simulink model "AUAV_V3_TestSensors"  (R2015a)
settings: Solver=FixedStepDiscrete  StartTime=0.0  StopTime=10.0  FixedStep=T  RelTol=1e-3
PreLoadFcn:
  | %T = 0.0025;
  | MavlinkBus;
  | mcuInit;
  | % Baro Altitude Computation
  | % =========================
  | basePressure = 98192.64;
  | baseTemp = 288.215;
  | lapseRate = -0.00198122;
  | baseHeight = 0;
undefined symbols (not defined in the file): A0, A14, A15, A2, A3, A4, A5, A6, accBiasRateLimit, apSampleTime, B0, bankCommandLimit, barAdjust, baroCutoff, baroCutTemp, baroOffset, baroScale, barTGain1, barTGain2, barTMean1, barTMean2, bda, bde, bdr, bdt, bICda, bICde, bICdr, bICdt, cubeAccelGain16405, cubeGyroGain16405, cubeMagGain16405, D0, D11, D7, D8, daLimit, data, daTrimMax, daTrimMin, deLimit, derivativesConstant, deTrimMax, deTrimMin, drLimit, drTrimMax, drTrimMin, dtLimit, dtTrimMax, dtTrimMin, F2, F3, G0, G13, G15, gaind, GS_location, gyroBiasRateLimit, IC1max, imuOffset_xacc ... (+77)
libraries: MCHP_Blockset x158, simulink x84, SLUGS_Library x31, aerolibconvert2 x6, aerolibutil x4, aerolibtransform2 x3, dspmtrx3 x2, aerolibobsolete x2
(part 20 of 23)

== system AUAV_V3_TestSensors/Inner Loop// Navigation/Longitudinal Channel Encaps [updated 4.28.16]/Longitudinal Channel/Height Error to Pitch Command [PI]/Trapezoidal Integrator ==
  x : Inport
  Reset : Inport  Port=2
  Constant : Constant  Value=1/3  OutDataTypeStr=single
  Constant1 : Constant  Value=4/3  OutDataTypeStr=single
  Constant2 : Constant  Value=T/2  OutDataTypeStr=single
  Constant3 : Constant  Value=1/3  OutDataTypeStr=single
  Constant5 : Constant  Value=0  OutDataTypeStr=single
  Integer Delay : Delay  DelayLength=1  InputProcessing=Inherited  SampleTime=T
  Integer Delay1 : Delay  InputProcessing=Inherited  SampleTime=T
  Integer Delay2 : Delay  DelayLength=1  InputProcessing=Inherited  SampleTime=T
  Product{,1..3} (4 alike) : Product  OutDataTypeStr=single  RndMeth=Zero
  Protect NaNs : Subsystem
  "Protect NaNs " : Subsystem
  Subtract : Sum  Inputs=3  OutDataTypeStr=single
  Subtract1 : Sum  Inputs=2  OutDataTypeStr=single
  Switch1 : Switch  Criteria=u2 > Threshold  Threshold=0.3  SampleTime=.01
  Int(x) : Outport
  wires:
  Constant/1 -> Product/2
  Constant1/1 -> Product1/2
  Integer Delay/1 -> Product1/1
  Integer Delay1/1 -> Product2/1
  Constant3/1 -> Product2/2
  x/1 -> "Protect NaNs "/1(In1)
  Product/1 -> Subtract/1
  Product1/1 -> Subtract/2
  Product2/1 -> Subtract/3
  Constant2/1 -> Product3/1
  Subtract/1 -> Product3/2
  Subtract1/1 -> Switch1/3
  Integer Delay2/1 -> Subtract1/1
  Product3/1 -> Subtract1/2
  Constant5/1 -> Switch1/1
  Reset/1 -> Switch1/2
  Switch1/1 -> Protect NaNs/1(In1)
  Protect NaNs/1(Out1) -> Int(x)/1, Integer Delay2/1
  "Protect NaNs "/1(Out1) -> Product/1, Integer Delay/1, Integer Delay1/1

== system AUAV_V3_TestSensors/Inner Loop// Navigation/Longitudinal Channel Encaps [updated 4.28.16]/Longitudinal Channel/Pitch To Elevator [PID]/Trapezoidal Integrator ==
  x : Inport
  Reset : Inport  Port=2
  Constant : Constant  Value=1/3  OutDataTypeStr=single
  Constant1 : Constant  Value=4/3  OutDataTypeStr=single
  Constant2 : Constant  Value=T/2  OutDataTypeStr=single
  Constant3 : Constant  Value=1/3  OutDataTypeStr=single
  Constant5 : Constant  Value=0  OutDataTypeStr=single
  Integer Delay : Delay  DelayLength=1  InputProcessing=Inherited  SampleTime=T
  Integer Delay1 : Delay  InputProcessing=Inherited  SampleTime=T
  Integer Delay2 : Delay  DelayLength=1  InputProcessing=Inherited  SampleTime=T
  Product{,1..3} (4 alike) : Product  OutDataTypeStr=single  RndMeth=Zero
  "Protect NaNs " : Subsystem
  Protect NaNs1 : Subsystem
  Subtract : Sum  Inputs=3  OutDataTypeStr=single
  Subtract1 : Sum  Inputs=2  OutDataTypeStr=single
  Switch1 : Switch  Criteria=u2 > Threshold  Threshold=0.3  SampleTime=.01
  Int(x) : Outport
  wires:
  Switch1/1 -> Protect NaNs1/1(In1)
  Reset/1 -> Switch1/2
  Constant5/1 -> Switch1/1
  Product3/1 -> Subtract1/2
  Integer Delay2/1 -> Subtract1/1
  Subtract1/1 -> Switch1/3
  Subtract/1 -> Product3/2
  Constant2/1 -> Product3/1
  Product2/1 -> Subtract/3
  Product1/1 -> Subtract/2
  Product/1 -> Subtract/1
  x/1 -> "Protect NaNs "/1(In1)
  Constant3/1 -> Product2/2
  Integer Delay1/1 -> Product2/1
  Integer Delay/1 -> Product1/1
  Constant1/1 -> Product1/2
  Constant/1 -> Product/2
  Protect NaNs1/1(Out1) -> Integer Delay2/1, Int(x)/1
  "Protect NaNs "/1(Out1) -> Integer Delay1/1, Integer Delay/1, Product/1

== system AUAV_V3_TestSensors/Inner Loop// Navigation/Longitudinal Channel Encaps [updated 4.28.16]/Longitudinal Channel/Pitot Control End/ 0.3 sec tau for high speeds ==
  In1 : Inport
  Constant : Constant  Value=T
  Constant1 : Constant  Value=f
  Embedded MATLAB Function : MATLAB Function  TreatAsAtomicUnit=on
  Out1 : Outport
  wires:
  Constant/1 -> Embedded MATLAB Function/2(T)
  Constant1/1 -> Embedded MATLAB Function/3(f)
  Embedded MATLAB Function/1(y) -> Out1/1
  In1/1 -> Embedded MATLAB Function/1(u)

== system AUAV_V3_TestSensors/Inner Loop// Navigation/Longitudinal Channel Encaps [updated 4.28.16]/Longitudinal Channel/Pitot Control End/Air Density from Height ==
  h(m) : Inport
  Add : Sum  Inputs=+-
  Constant : Constant  OutDataTypeStr=single
  Constant 2 from Model : Constant  Value=4.255876  OutDataTypeStr=single
  Constant from Model : Constant  Value=145442  OutDataTypeStr=single
  Divide : Product  Inputs=*/
  Divide1 : Product
  Length Conversion : aerolibconvert2/Length Conversion  IU=m  OU=ft
  Rho_0 (Kg/m^3) : Constant  Value=1.225  OutDataTypeStr=single
  "[0 1000]" : Saturate  UpperLimit=1000  LowerLimit=0
  dsPIC Power : Subsystem  AncestorBlock=SLUGS_Library/dsPIC Power
  rho (Kg/m^3) : Outport
  wires:
  Constant/1 -> Add/1
  Divide/1 -> Add/2
  h(m)/1 -> "[0 1000]"/1
  Constant from Model/1 -> Divide/2
  Rho_0 (Kg/m^3)/1 -> Divide1/2
  Divide1/1 -> rho (Kg/m^3)/1
  Length Conversion/1 -> Divide/1
  Add/1 -> dsPIC Power/1(u)
  Constant 2 from Model/1 -> dsPIC Power/2(v)
  dsPIC Power/1(u^v) -> Divide1/1
  "[0 1000]"/1 -> Length Conversion/1

== system AUAV_V3_TestSensors/Inner Loop// Navigation/Longitudinal Channel Encaps [updated 4.28.16]/Longitudinal Channel/Pitot Control End/Compute Airspeed ==
  Dyn P : Inport
  rho : Inport  Port=2
  Divide2 : Product  Inputs=**/
  "[ 0.01 50000]" : Saturate  UpperLimit=50000  LowerLimit=0.01
  a : Constant  Value=2  OutDataTypeStr=single
  dsPIC_SQRT : Subsystem  AncestorBlock=SLUGS_Library/dsPIC_SQRT
  Airspeed m(s) : Outport
  wires:
  "[ 0.01 50000]"/1 -> Divide2/3
  rho/1 -> "[ 0.01 50000]"/1
  Dyn P/1 -> Divide2/2
  a/1 -> Divide2/1
  dsPIC_SQRT/1(sqrt(x)) -> Airspeed m(s)/1
  Divide2/1 -> dsPIC_SQRT/1(x)

== system AUAV_V3_TestSensors/Inner Loop// Navigation/Longitudinal Channel Encaps [updated 4.28.16]/Longitudinal Channel/Pitot Control End/Protect NaN ==
  In1 : Inport
  Integer Delay3 : Delay  DelayLength=1  InputProcessing=Inherited  SampleTime=T
  Relational Operator2 : RelationalOperator  Operator===  OutDataTypeStr=uint(8)
  Switch3 : Switch  Criteria=u2 > Threshold  Threshold=0.3  SampleTime=.01
  Out1 : Outport
  wires:
  Integer Delay3/1 -> Switch3/3
  Switch3/1 -> Out1/1, Integer Delay3/1
  In1/1 -> Relational Operator2/2, Relational Operator2/1, Switch3/1
  Relational Operator2/1 -> Switch3/2

== system AUAV_V3_TestSensors/Inner Loop// Navigation/Navigation Encaps [updated 4.28.16]/Navigation/Circle Navigation/Get SP Location ==
  GS LLA : Inport
  GS R_in : Inport  Port=2
  ISR Location : Inport  Port=3
  Demux : Demux  Outputs=3
  Geod2LTP : SLUGS_Library/Navigation/Geod2LTP
  Integer Delay1 : Delay  DelayLength=1  InputProcessing=Inherited
  Selector : Selector  InputPortWidth=3  Indices=[3]
  Zero out Z2 : MATLAB Function  TreatAsAtomicUnit=on
  Hc : Outport
  SP : Outport  Port=2
  wires:
  Integer Delay1/1 -> Hc/1
  Selector/1 -> Integer Delay1/1
  Zero out Z2/1(P) -> SP/1
  Geod2LTP/1 -> Selector/1, Zero out Z2/1(Pin)
  GS LLA/1 -> Geod2LTP/1
  Demux/3 -> Geod2LTP/5
  Demux/2 -> Geod2LTP/4
  Demux/1 -> Geod2LTP/3
  GS R_in/1 -> Geod2LTP/2
  ISR Location/1 -> Demux/1

== system AUAV_V3_TestSensors/Inner Loop// Navigation/Navigation Encaps [updated 4.28.16]/Navigation/Circle Navigation/Inside the Circle, Keep Straight until intersection ==
  ISR Loc : Inport
  R : Inport  Port=2
  Puav : Inport  Port=3
  Action Port : ActionPort  ActionType=elseif
  Compute Head of Circle : MATLAB Function  TreatAsAtomicUnit=on
  RTB1 : Constant  OutDataTypeStr=uint8
  Subtract : Sum  Inputs=+-  OutDataTypeStr=single
  L2 Vec : Outport
  Mode : Outport  Port=2
  wires:
  RTB1/1 -> Mode/1
  R/1 -> Compute Head of Circle/1(R)
  ISR Loc/1 -> Compute Head of Circle/2(ISR)
  Compute Head of Circle/1(topCoord) -> Subtract/1
  Puav/1 -> Subtract/2
  Subtract/1 -> L2 Vec/1

== system AUAV_V3_TestSensors/Inner Loop// Navigation/Navigation Encaps [updated 4.28.16]/Navigation/Circle Navigation/Intersection. Circular Navigation ==
  R : Inport
  L2 : Inport  Port=2
  d : Inport  Port=3
  ISR Loc : Inport  Port=4
  UAV m ISR : Inport  Port=5
  Vxyz : Inport  Port=6
  |Vg| : Inport  Port=7
  Puav : Inport  Port=8
  Action Port : ActionPort  ActionType=else
  Compute Angle Between Vectors1 : Subsystem  AncestorBlock=SLUGS_Library/Compute Angle Between Vectors
  Compute Angle Between Vectors2 : Subsystem  AncestorBlock=SLUGS_Library/Compute Angle Between Vectors
  Embedded MATLAB Function : MATLAB Function  TreatAsAtomicUnit=on
  Product{,1..2,4..5,7} (6 alike) : Product  RndMeth=Zero
  Product3 : Product  Inputs=*/  RndMeth=Zero
  Product6 : Product  Inputs=*/  RndMeth=Zero
  RTB1 : Constant  Value=2  OutDataTypeStr=uint8
  Relational Operator : RelationalOperator  Operator=<=  OutDataTypeStr=boolean
  Subtract : Sum  Inputs=+-+
  Subtract1 : Sum  Inputs=2
  Subtract2 : Sum  Inputs=+-
  Subtract3 : Sum  Inputs=2
  Subtract5 : Sum  Inputs=+-
  Subtract6 : Sum  Inputs=-+
  Switch1 : Switch  Criteria=u2 > Threshold  Threshold=0.3  ZeroCross=off
  "d " : InportShadow  Port=3
  dsPIC_ABS : Subsystem  AncestorBlock=SLUGS_Library/dsPIC_ABS
  dsPIC_ABS1 : Subsystem  AncestorBlock=SLUGS_Library/dsPIC_ABS
  dsPIC_SQRT : Subsystem  AncestorBlock=SLUGS_Library/dsPIC_SQRT
  negprotect1 : MATLAB Function  TreatAsAtomicUnit=on
  negprotect2 : MATLAB Function  TreatAsAtomicUnit=on
  L2 Vec : Outport
  Mode : Outport  Port=2
  wires:
  R/1 -> Product/1, Product/2
  L2/1 -> Product1/1, Product1/2
  d/1 -> Product2/1, Product2/2, Subtract1/1, Subtract1/2
  Product/1 -> Subtract/1, Subtract2/1  "r^2"
  Product1/1 -> Subtract/2
  Product2/1 -> Subtract/3
  Subtract/1 -> Product3/1  "r^2 - L2^2 + d^2"
  negprotect2/1(zpVal) -> Product3/2  "2d"
  Subtract1/1 -> negprotect2/1(val)
  Product3/1 -> Product4/2, Product4/1, [a]  "a"
  Product4/1 -> Subtract2/2  "a^2"
  Subtract2/1 -> dsPIC_SQRT/1(x)  "h"
  negprotect1/1(zpVal) -> Product6/2  "d"
  "d "/1 -> negprotect1/1(val)
  ISR Loc/1 -> Subtract3/1
  Subtract3/1 -> Embedded MATLAB Function/2(P2)  "P2"
  UAV m ISR/1 -> Product6/1
  Product7/1 -> Subtract3/2
  Product6/1 -> Product7/1, [UavMIsDbd]
  [a] -> Product7/2
  [UavMIsDbd] -> Product5/2
  Vxyz/1 -> Compute Angle Between Vectors1/1(Vxyz), Compute Angle Between Vectors2/1(Vxyz)
  |Vg|/1 -> Compute Angle Between Vectors1/2(|Vg|), Compute Angle Between Vectors2/2(|Vg|)
  Compute Angle Between Vectors2/1(alpha) -> dsPIC_ABS1/1(x)
  dsPIC_ABS1/1(|x|) -> Relational Operator/1
  Compute Angle Between Vectors1/1(alpha) -> dsPIC_ABS/1(x)
  dsPIC_ABS/1(|x|) -> Relational Operator/2
  Relational Operator/1 -> Switch1/2
  RTB1/1 -> Mode/1
  dsPIC_SQRT/1(sqrt(x)) -> Product5/1  "h"
  Product5/1 -> Embedded MATLAB Function/1(hFact)
  Subtract5/1 -> Compute Angle Between Vectors2/3(P3), Switch1/1
  Embedded MATLAB Function/1(P31) -> Subtract5/1
  Subtract6/1 -> Compute Angle Between Vectors1/3(P3), Switch1/3
  Embedded MATLAB Function/2(P32) -> Subtract6/2
  Puav/1 -> Subtract5/2, Subtract6/1
  Switch1/1 -> L2 Vec/1

== system AUAV_V3_TestSensors/Inner Loop// Navigation/Navigation Encaps [updated 4.28.16]/Navigation/Circle Navigation/No intersection, Navigate to ISR ==
  Puav : Inport
  ISR Loc : Inport  Port=2
  Action Port : ActionPort  ActionType=then
  RTB1 : Constant  Value=0  OutDataTypeStr=uint8
  Subtract : Sum  Inputs=+-
  L2 Vec : Outport
  Mode : Outport  Port=2
  wires:
  ISR Loc/1 -> Subtract/1
  Puav/1 -> Subtract/2
  Subtract/1 -> L2 Vec/1
  RTB1/1 -> Mode/1

== system AUAV_V3_TestSensors/Inner Loop// Navigation/Navigation Encaps [updated 4.28.16]/Navigation/Circle Navigation/Vector Norm ==
  Vector : Inport
  dsPIC Dot Product : SLUGS_Library/dsPIC Dot Product
  dsPIC_SQRT : Subsystem  AncestorBlock=SLUGS_Library/dsPIC_SQRT
  Norm : Outport
  wires:
  dsPIC_SQRT/1(sqrt(x)) -> Norm/1
  Vector/1 -> dsPIC Dot Product/2, dsPIC Dot Product/1
  dsPIC Dot Product/1 -> dsPIC_SQRT/1(x)

== system AUAV_V3_TestSensors/Inner Loop// Navigation/Navigation Encaps [updated 4.28.16]/Navigation/Circle Navigation/dsPIC_ABS ==
  x : Inport
  Abs : Abs
  Environment Controller : simulink/Signal Routing/Environment Controller
  myAbs() apUtils.c [updated 5.1.16] : MCHP_Blockset/User Functions/C Function Call  ParseFilesChkbx=off  ListFunctions1=Custom Function  Function1=float myAbs(float x)  AddHeaderDeclaration=off  Function1Type=when block is updated (default)  Fct1BlockIn=x  FctReturnBlockOut=on  DataCollected=0  ORDERING=None  SampleTime=-1  MCHP_MASTERLINK=|  PinDigitalInput=[]  PinDigitalOutput=[]  PinAnalogInput=[]
      | AUAV_V3_TestSensors/Microchip Master
      | AUAV V3 Board
      | Busy Flag on D2 (RA6)
  |x| : Outport
  wires:
  Environment Controller/1 -> |x|/1
  Abs/1 -> Environment Controller/1
  myAbs() apUtils.c [updated 5.1.16]/1 -> Environment Controller/2
  x/1 -> Abs/1, myAbs() apUtils.c [updated 5.1.16]/1

== system AUAV_V3_TestSensors/Inner Loop// Navigation/Navigation Encaps [updated 4.28.16]/Navigation/Get 2D Groundspeed/Vector Norm ==
  Vector : Inport
  dsPIC Dot Product : SLUGS_Library/dsPIC Dot Product
  dsPIC_SQRT : Subsystem  AncestorBlock=SLUGS_Library/dsPIC_SQRT
  Norm : Outport
  wires:
  dsPIC_SQRT/1(sqrt(x)) -> Norm/1
  Vector/1 -> dsPIC Dot Product/2, dsPIC Dot Product/1
  dsPIC Dot Product/1 -> dsPIC_SQRT/1(x)

== system AUAV_V3_TestSensors/Inner Loop// Navigation/Navigation Encaps [updated 4.28.16]/Navigation/L2+/Get Sin, Cos eta ==
  |V_g| : Inport
  L2_vec : Inport  Port=2
  Vxyz : Inport  Port=3
  "2D Dot Product " : Subsystem
  Compare To Zero : simulink/Logic and Bit Operations/Compare To Zero  relop===  OutDataTypeStr=uint8  ZeroCross=off
  Dead Zone : DeadZone  LowerValue=-0.1  UpperValue=0.1  SaturateOnIntegerOverflow=on
  Display : Display
  Display1 : Display
  Divide1 : Product  Inputs=/*
  Divide2 : Product  Inputs=*/
  Get Groundspeed : Subsystem
  Get ZProd : Subsystem
  Product1 : Product  RndMeth=Zero
  Switch : Switch  Criteria=u2 > Threshold  Threshold=0.3  ZeroCross=off
  Switch2 : Switch  Criteria=u2 > Threshold  Threshold=0.3  ZeroCross=off
  cos(pi/2) : Constant  Value=0  OutDataTypeStr=single
  negprotect : MATLAB Function  TreatAsAtomicUnit=on
  sin(pi/2) : Constant  OutDataTypeStr=single
  sin(eta) : Outport
  cos(eta) : Outport  Port=2
  wires:
  negprotect/1(zpVal) -> Divide2/2, Divide1/1, Dead Zone/1
  Switch/1 -> Display/1, sin(eta)/1
  Divide2/1 -> Switch/3
  Get ZProd/1(Z_prod) -> Divide2/1
  Divide1/1 -> Switch2/3
  cos(pi/2)/1 -> Switch2/1
  Switch2/1 -> Display1/1, cos(eta)/1
  sin(pi/2)/1 -> Switch/1
  "2D Dot Product "/1(2D _dot) -> Divide1/2
  Product1/1 -> negprotect/1(val)
  |V_g|/1 -> Product1/2
  Get Groundspeed/1(|L2|) -> Product1/1
  Vxyz/1 -> "2D Dot Product "/1(Vxyz), Get ZProd/2(Vxyz)
  L2_vec/1 -> Get Groundspeed/1(L2_vec), "2D Dot Product "/2(L2_vec), Get ZProd/1(L2_vec)
  Dead Zone/1 -> Compare To Zero/1
  Compare To Zero/1 -> Switch2/2, Switch/2

== system AUAV_V3_TestSensors/Inner Loop// Navigation/Navigation Encaps [updated 4.28.16]/Navigation/L2+/L2+ ==
  sin(eta) : Inport
  |V_g| : Inport  Port=2
  T* : Inport  Port=3
  Display3 : Display
  Divide : Product  Inputs=**/
  Gain : Gain  Gain=2  SampleTime=0.01
  negprotect : MATLAB Function  TreatAsAtomicUnit=on
  a_c : Outport
  wires:
  T*/1 -> negprotect/1(val)
  Gain/1 -> Display3/1, a_c/1
  |V_g|/1 -> Divide/2
  Divide/1 -> Gain/1
  sin(eta)/1 -> Divide/1
  negprotect/1(zpVal) -> Divide/3

== system AUAV_V3_TestSensors/Inner Loop// Navigation/Navigation Encaps [updated 4.28.16]/Navigation/L2+/Subsystem ==
  a_c : Inport
  Bank  Limit Command : Saturate  UpperLimit=bankCommandLimit  LowerLimit=-bankCommandLimit  SampleTime=apSampleTime
  Constant : Constant  Value=ISA_g  OutDataTypeStr=single
  Product : Product  Inputs=*/  RndMeth=Zero
  To Workspace3 : ToWorkspace  VariableName=Phic  SampleTime=-1
  dsPIC_atan : Subsystem  AncestorBlock=SLUGS_Library/dsPIC_atan
  phi_c : Outport
  wires:
  Bank  Limit Command/1 -> To Workspace3/1, phi_c/1
  dsPIC_atan/1(atan(x)) -> Bank  Limit Command/1
  Product/1 -> dsPIC_atan/1(x)
  Constant/1 -> Product/2
  a_c/1 -> Product/1

== system AUAV_V3_TestSensors/Inner Loop// Navigation/Navigation Encaps [updated 4.28.16]/Navigation/L2+/dsPIC_ABS ==
  x : Inport
  Abs : Abs
  Environment Controller : simulink/Signal Routing/Environment Controller
  myAbs() apUtils.c [updated 5.1.16] : MCHP_Blockset/User Functions/C Function Call  ParseFilesChkbx=off  ListFunctions1=Custom Function  Function1=float myAbs(float x)  AddHeaderDeclaration=on  Function1Type=when block is updated (default)  Fct1BlockIn=x  FctReturnBlockOut=on  DataCollected=0  ORDERING=None  SampleTime=-1  MCHP_MASTERLINK=|  PinDigitalInput=[]  PinDigitalOutput=[]  PinAnalogInput=[]
      | AUAV_V3_TestSensors/Microchip Master
      | AUAV V3 Board
      | Busy Flag on D2 (RA6)
  |x| : Outport
  wires:
  Environment Controller/1 -> |x|/1
  Abs/1 -> Environment Controller/1
  myAbs() apUtils.c [updated 5.1.16]/1 -> Environment Controller/2
  x/1 -> Abs/1, myAbs() apUtils.c [updated 5.1.16]/1

== system AUAV_V3_TestSensors/Inner Loop// Navigation/Navigation Encaps [updated 4.28.16]/Navigation/L2+/dsPIC_atan2 ==
  u : Inport
  v : Inport  Port=2
  Environment Controller : simulink/Signal Routing/Environment Controller
  Trigonometric Function : Trigonometry  Operator=atan2
  myAtan2() apUtils.c [updated 5.1.16] : MCHP_Blockset/User Functions/C Function Call  ParseFilesChkbx=off  ListFunctions1=Custom Function  Function1=float myAtan2(float num, float denom)  AddHeaderDeclaration=on  Function1Type=when block is updated (default)  Fct1BlockIn="num  , denom"  FctReturnBlockOut=on  DataCollected=0  ORDERING=None  SampleTime=-1  MCHP_MASTERLINK=|  PinDigitalInput=[]  PinDigitalOutput=[]  PinAnalogInput=[]
      | AUAV_V3_TestSensors/Microchip Master
      | AUAV V3 Board
      | Busy Flag on D2 (RA6)
  atan2(x,y) : Outport
  wires:
  Environment Controller/1 -> atan2(x,y)/1
  myAtan2() apUtils.c [updated 5.1.16]/1 -> Environment Controller/2
  Trigonometric Function/1 -> Environment Controller/1
  v/1 -> Trigonometric Function/2, myAtan2() apUtils.c [updated 5.1.16]/2
  u/1 -> Trigonometric Function/1, myAtan2() apUtils.c [updated 5.1.16]/1

== system AUAV_V3_TestSensors/Inner Loop// Navigation/Navigation Encaps [updated 4.28.16]/Navigation/L2+/if sin(eta) < 0 - maxAcc else maxAcc  ==
  sin(eta) : Inport
  Compare To Zero : simulink/Logic and Bit Operations/Compare To Zero  relop=<  OutDataTypeStr=uint8  ZeroCross=off
  Constant1 : Constant  Value=maxAcc  OutDataTypeStr=single
  Constant9 : Constant  Value=-maxAcc  OutDataTypeStr=single
  Switch1 : Switch  Criteria=u2 > Threshold  Threshold=0.3
  + - maxAcc : Outport
  wires:
  Switch1/1 -> + - maxAcc/1
  sin(eta)/1 -> Compare To Zero/1
  Constant1/1 -> Switch1/3
  Constant9/1 -> Switch1/1
  Compare To Zero/1 -> Switch1/2

== system AUAV_V3_TestSensors/Inner Loop// Navigation/Navigation Encaps [updated 4.28.16]/Navigation/Line Segment/Vector Norm ==
  Vector : Inport
  dsPIC Dot Product : SLUGS_Library/dsPIC Dot Product
  dsPIC_SQRT : Subsystem  AncestorBlock=SLUGS_Library/dsPIC_SQRT
  Norm : Outport
  wires:
  dsPIC_SQRT/1(sqrt(x)) -> Norm/1
  Vector/1 -> dsPIC Dot Product/2, dsPIC Dot Product/1
  dsPIC Dot Product/1 -> dsPIC_SQRT/1(x)

== system AUAV_V3_TestSensors/Inner Loop// Navigation/Navigation Encaps [updated 4.28.16]/Navigation/Normal WP Navigation/Compute WP Switching Trigger ==
  ToWp : Inport
  T1 : Inport  Port=2
  N1 : Inport  Port=3
  LeadDistance : Inport  Port=4
  Puav : Inport  Port=5
  L2 : Inport  Port=6
  Add : Sum  Inputs=+-
  Add1 : Sum  Inputs=+-
  Add3 : Sum  Inputs=--
  Compute Projection : Subsystem
  Constant1 : Constant  Value=0  OutDataTypeStr=single
  Constant3 : Constant  Value=MaxDwnPthStar  OutDataTypeStr=single
  Constant4 : Constant  Value=tanIntercept  OutDataTypeStr=single
  Divide : Product  Inputs=*/
  Divide1 : Product
  Product : Product  RndMeth=Zero
  Product1 : Product  RndMeth=Zero
  Product2 : Product  RndMeth=Zero
  "Puav " : InportShadow  Port=5
  Relational Operator : RelationalOperator  Operator=>  OutDataTypeStr=boolean
  Subtract : Sum  Inputs=+-  OutDataTypeStr=single
  Switch Distance Less than? : RelationalOperator  Operator=<  OutDataTypeStr=uint(8)  SampleTime=apSampleTime
  Switch1 : Switch  Criteria=u2 > Threshold  Threshold=0.3
  "T1 " : InportShadow  Port=2
  "WP1 " : InportShadow
  dsPIC Dot Product : SLUGS_Library/dsPIC Dot Product
  dsPIC_ABS : Subsystem  AncestorBlock=SLUGS_Library/dsPIC_ABS
  dsPIC_SQRT : Subsystem  AncestorBlock=SLUGS_Library/dsPIC_SQRT
  max : SLUGS_Library/max
  max1 : SLUGS_Library/max
  min : SLUGS_Library/min
  Switch : Outport
  Dist2WP1 : Outport  Port=2
  L2Vec : Outport  Port=3
  wires:
  Puav/1 -> Compute Projection/1(Pned)
  Compute Projection/1(D2wp1) -> Switch Distance Less than?/1, Dist2WP1/1, [Dwp1]
  LeadDistance/1 -> Switch Distance Less than?/2
  ToWp/1 -> Compute Projection/2(ToWp)
  T1/1 -> Compute Projection/3(T)
  Switch Distance Less than?/1 -> Switch/1
  "Puav "/1 -> Subtract/1
  "WP1 "/1 -> Subtract/2
  Subtract/1 -> dsPIC Dot Product/1, [Pwp1]
  dsPIC Dot Product/1 -> dsPIC_ABS/1(x)  "e_N"
  dsPIC_ABS/1(|x|) -> Divide/1, [abs_e_N]
  Constant4/1 -> Divide/2
  Divide/1 -> min/2  "|e_N|/tanInt"
  L2/1 -> Divide1/1, [L2]
  Constant3/1 -> Divide1/2
  Divide1/1 -> min/1
  min/1 -> max1/1, Switch1/1  "minDownPath"
  Relational Operator/1 -> Switch1/2
  [L2] -> Relational Operator/2
  [abs_e_N] -> Relational Operator/1
  Switch1/1 -> Add1/2  "L2DownPath"
  Add/1 -> dsPIC_SQRT/1(x)
  dsPIC_SQRT/1(sqrt(x)) -> max1/2
  [L2] -> Product/1, Product/2
  Product/1 -> Add/1
  [abs_e_N] -> Product1/2, Product1/1
  Product1/1 -> Add/2
  max1/1 -> Switch1/3
  [Dwp1] -> Add1/1
  Add1/1 -> max/1
  Constant1/1 -> max/2
  max/1 -> Product2/1
  "T1 "/1 -> Product2/2
  Product2/1 -> Add3/1
  [Pwp1] -> Add3/2
  Add3/1 -> L2Vec/1
  N1/1 -> dsPIC Dot Product/2

== system AUAV_V3_TestSensors/Inner Loop// Navigation/Navigation Encaps [updated 4.28.16]/Navigation/Normal WP Navigation/Get Frenet ==
  GS LLA : Inport
  GS R_in : Inport  Port=2
  From WP : Inport  Port=3
  To WP : Inport  Port=4
  TurnLeadTime : Inport  Port=5
  |V_g| : Inport  Port=6
  Enable : EnablePort
  Compute Frenet : Subsystem  AncestorBlock=SLUGS_Library/Navigation/Compute Frenet
  Demux1 : Demux  Outputs=3
  GS LLA_1 : InportShadow
  GS R_in_1 : InportShadow  Port=2
  Integer Delay1 : Delay  DelayLength=1  InitialCondition=1  InputProcessing=Inherited
  Product1 : Product  OutDataTypeStr=single  RndMeth=Zero
  Terminator1 : Terminator
  Terminator2 : Terminator
  To Workspace2 : ToWorkspace  VariableName=fromWP  SampleTime=-1
  To Workspace3 : ToWorkspace  VariableName=toWP  SampleTime=-1
  Zero out Z1 : MATLAB Function  TreatAsAtomicUnit=on
  Zero out Z2 : MATLAB Function  TreatAsAtomicUnit=on
  Zero out Z3 : MATLAB Function  TreatAsAtomicUnit=on
  get WP Coord from Index1 : Subsystem  AncestorBlock=SLUGS_Library/Navigation/get WP Coord from Index
  get WP Coord from Index2 : Subsystem  AncestorBlock=SLUGS_Library/Navigation/get WP Coord from Index
  H_c : Outport
  ToWp : Outport  Port=2
  T1 : Outport  Port=3
  N1 : Outport  Port=4
  TurnLeadDistance : Outport  Port=5
  wires:
  Zero out Z3/1(P) -> ToWp/1
  Integer Delay1/1 -> H_c/1
  Compute Frenet/2(N) -> Zero out Z1/1(Pin)
  Demux1/3 -> Integer Delay1/1
  Compute Frenet/1(T) -> Zero out Z2/1(Pin)
  |V_g|/1 -> Product1/2
  TurnLeadTime/1 -> Product1/1
  Product1/1 -> TurnLeadDistance/1
  Zero out Z2/1(P) -> T1/1
  Zero out Z1/1(P) -> N1/1
  get WP Coord from Index1/1(WP Coord) -> Compute Frenet/1(Pos 1), To Workspace2/1
  get WP Coord from Index2/1(WP Coord) -> Demux1/1, Compute Frenet/2(Pos 2), To Workspace3/1, Zero out Z3/1(Pin)
  From WP/1 -> get WP Coord from Index1/1(WP Idx)
  GS LLA/1 -> get WP Coord from Index1/2(GS LLA)
  GS R_in/1 -> get WP Coord from Index1/3(GS R_in)
  To WP/1 -> get WP Coord from Index2/1(WP Idx)
  GS LLA_1/1 -> get WP Coord from Index2/2(GS LLA)
  GS R_in_1/1 -> get WP Coord from Index2/3(GS R_in)
  Demux1/1 -> Terminator2/1
  Demux1/2 -> Terminator1/1

== system AUAV_V3_TestSensors/Inner Loop// Navigation/Navigation Encaps [updated 4.28.16]/Navigation/Normal WP Navigation/On WP Enable ==
  L2 : Inport
  GS LLA : Inport  Port=2
  GS R_in : Inport  Port=3
  Enable : EnablePort
  Constant5 : Constant  Value=IPStar  OutDataTypeStr=single
  Product : Product  Inputs=3  RndMeth=Zero
  Subsystem : Subsystem
  Subtract : Sum  Inputs=+-
  P_i : Outport
  wires:
  Constant5/1 -> Product/3
  L2/1 -> Product/1
  Product/1 -> Subtract/2
  Subtract/1 -> P_i/1  "WP0 - L2*IP*T1"
  GS LLA/1 -> Subsystem/1(GS LLA)
  GS R_in/1 -> Subsystem/2(GS R_in)
  Subsystem/2(T1) -> Product/2
  Subsystem/1(WP0) -> Subtract/1

== system AUAV_V3_TestSensors/Inner Loop// Navigation/Navigation Encaps [updated 4.28.16]/Navigation/Normal WP Navigation/Vector Norm ==
  Vector : Inport
  dsPIC Dot Product : SLUGS_Library/dsPIC Dot Product
  dsPIC_SQRT : Subsystem  AncestorBlock=SLUGS_Library/dsPIC_SQRT
  Norm : Outport
  wires:
  dsPIC_SQRT/1(sqrt(x)) -> Norm/1
  Vector/1 -> dsPIC Dot Product/2, dsPIC Dot Product/1
  dsPIC Dot Product/1 -> dsPIC_SQRT/1(x)

== system AUAV_V3_TestSensors/Inner Loop// Navigation/Navigation Encaps [updated 4.28.16]/Navigation/RTB//Follow Mobile Navigation/Compute Mobile Location ==
  "Lat, Lon" : Inport
  GS LLA : Inport  Port=2
  GS R : Inport  Port=3
  Enable : EnablePort  StatesWhenEnabling=reset
  Demux4 : Demux  Outputs=2
  Geod2LTP : SLUGS_Library/Navigation/Geod2LTP
  No Height All in 2D : Constant  Value=0  OutDataTypeStr=single
  XYZ : Outport
  wires:
  Geod2LTP/1 -> XYZ/1
  "Lat, Lon"/1 -> Demux4/1
  Demux4/2 -> Geod2LTP/4
  Demux4/1 -> Geod2LTP/3
  No Height All in 2D/1 -> Geod2LTP/5
  GS R/1 -> Geod2LTP/2
  GS LLA/1 -> Geod2LTP/1

== system AUAV_V3_TestSensors/Inner Loop// Navigation/Navigation Encaps [updated 4.28.16]/Navigation/RTB//Follow Mobile Navigation/Simple Predictor ==
  Base Point : Inport
  Discrete-Time Integrator : DiscreteIntegrator  InitialConditionSource=external  SampleTime=0.01
  Gain : Gain
  Gain1 : Gain  Gain=3
  Sum : Sum  Inputs=|+-
  Sum1 : Sum  Inputs=++|
  Predicted Bp : Outport
  wires:
  Discrete-Time Integrator/1 -> Gain/1
  Sum/1 -> Gain1/1, Discrete-Time Integrator/1
  Gain/1 -> Sum/2, Sum1/2
  Gain1/1 -> Sum1/1
  Base Point/1 -> Sum/1, Discrete-Time Integrator/2
  Sum1/1 -> Predicted Bp/1

== system AUAV_V3_TestSensors/Inner Loop// Navigation/Navigation Encaps [updated 4.28.16]/Navigation/RTB//Follow Mobile Navigation/Vector Norm ==
  Vector : Inport
  dsPIC Dot Product : SLUGS_Library/dsPIC Dot Product
  dsPIC_SQRT : Subsystem  AncestorBlock=SLUGS_Library/dsPIC_SQRT
  Norm : Outport
  wires:
  dsPIC_SQRT/1(sqrt(x)) -> Norm/1
  Vector/1 -> dsPIC Dot Product/2, dsPIC Dot Product/1
  dsPIC Dot Product/1 -> dsPIC_SQRT/1(x)

== system AUAV_V3_TestSensors/Inner Loop// Navigation/Navigation Encaps [updated 4.28.16]/Navigation/Recent Enable/Grab Upon Enable ==
  Enable : EnablePort
  Compute GS Location : Subsystem
  Constant : Constant  Value=GS_location  OutDataTypeStr=single
  Constant1 : Constant  Value=[0 36.988506 -122.055308]  OutDataTypeStr=single
  Data Type Conversion : DataTypeConversion  OutDataTypeStr=single
  Data Type Conversion1 : DataTypeConversion  OutDataTypeStr=single
  Data Type Conversion2 : DataTypeConversion  OutDataTypeStr=single
  Demux : Demux  Outputs=[1 2]
  Environment Controller : simulink/Signal Routing/Environment Controller
  Gain : Gain  Gain=0.001
  Gain1 : Gain  Gain=0.0000001
  Gain2 : Gain  Gain=0.0000001
  Get GS Location : DataStoreRead  DialogController=Simulink.DDGSource  DataStoreName=mlGSLocationFloat  DataStoreElements=mlGSLocationFloat.alt#mlGSLocationFloat.lat#mlGSLocationFloat.lon
  Mux : Mux  Inputs=3
  Terminator : Terminator
  Terminator1 : Terminator
  "GS, Lon, Lat" : Outport
  GS R_in : Outport  Port=2
  GS Altitude (m) : Outport  Port=3
  wires:
  Demux/2 -> Terminator/1
  Demux/1 -> GS Altitude (m)/1
  Compute GS Location/2(R_in) -> Data Type Conversion1/1
  Compute GS Location/1("Lon, Lat") -> Data Type Conversion/1
  Data Type Conversion/1 -> "GS, Lon, Lat"/1
  Data Type Conversion1/1 -> GS R_in/1
  Constant/1 -> Environment Controller/1
  Environment Controller/1 -> Compute GS Location/1(GS Location), Demux/1
  Constant1/1 -> Terminator1/1
  Get GS Location/1 -> Gain/1
  Get GS Location/2 -> Gain1/1
  Get GS Location/3 -> Gain2/1
  Mux/1 -> Data Type Conversion2/1
  Data Type Conversion2/1 -> Environment Controller/2
  Gain/1 -> Mux/1
  Gain1/1 -> Mux/2
  Gain2/1 -> Mux/3

== system AUAV_V3_TestSensors/Inner Loop// Navigation/Navigation Encaps [updated 4.28.16]/Navigation/Recent Enable/Subsystem ==
  WP Fly : Inport
  Data Type Conversion2 : DataTypeConversion  OutDataTypeStr=uint8  SampleTime=apSampleTime
  Detect Rising Edge : Subsystem
  Just Enab : Outport
  wires:
  WP Fly/1 -> Detect Rising Edge/1(In1)
  Detect Rising Edge/1(Out1) -> Data Type Conversion2/1
  Data Type Conversion2/1 -> Just Enab/1

== system AUAV_V3_TestSensors/Position_and_Attitude_Filter/Attitude Complimentary Filter COG/Normalize Vector1/Norm/Subsystem2 ==
  x : Inport
  "[apUtils.c]" : MCHP_Blockset/User Functions/C Function Call  ParseFilesChkbx=on  ListFunctions1=Custom Function  Function1=real32_T mySqrt(real32_T u1);  AddHeaderDeclaration=on  Function1Type=when block is updated (default)  FctReturnBlockOut=on  DataCollected="s.chksm=reshape({ '360325-Apr-2016 19:19:45','638502-Mar-2016 19:06:13','219625-Apr-2016 19:38:33','1593925-Apr-2016 19:41:14','3277826-Apr-2016 00:33:15','294426-Apr-2016 00:47:59','556001-Oct-2014 14:05:42','963201-Apr-2016 12:47:40','358819-Apr-2016 01:35:18','985925-Apr-2016 19:19:45'},1,10);s.File1=reshape({ '  float  myAtan2(float num, float denom)','  float  myPow(float x, float toTheN)','  float  mySqrt(float x)','  float  myAbs(float x)','  float  myAtan(float x)','  float  myAsin(float x)','  float  mySin(float x)','  float  myCos(float x)','  float  myTan(float x)','  float  myAcos(float x)','  float  myExp(float x)','  void  hugeDelay(void)','  void  smallDelay(void)','  void  tinyDelay(void)','  void  printToUart2(const char *fmt, ...)'},1,15);s.File2=reshape({ '  void  newCircBuffer(CBRef cB)','  void  freeCircBuffer(CBRef* cB)','  void  freeCircBuffer(CBRef* cB)',' unsigned int  getLength(CBRef cB)','  int  readHead(CBRef cB)','  int  readTail(CBRef cB)',' unsigned char  peak(CBRef cB)',' unsigned char  readFront(CBRef cB)',' unsigned char  writeBack(CBRef cB, unsigned char data)','  void  makeEmpty(CBRef cB)','  void  printCircBuf(CBRef cB)'},1,11);s.File3=reshape({ '  void  uartBufferInit(void)','  void  __attribute__((__interrupt__, no_auto_psv)) _U4RXInterrupt(void)','  void  getGPSRawData(unsigned char* gpsBuffer)',' unsigned char  isGPSNovatel(void)'},1,4);s.File4=reshape({ '  char  hex2char(char halfhex)','  float  degMinToDeg(unsigned char degrees, float minutes)',' unsigned char  gpsUbloxSeparate(unsigned char* outStream)','  void  gpsUbloxParse(void)','  void  getGpsUbloxMainData(float* data)','  char  gpSmbl(char symbl)',' unsigned char  myTokenizer(char* stringToTokenize, char token, char * returnToken)','  void  parseRMC(unsigned char* stream)','  void  parseGGA(unsigned char* stream)',' unsigned char  getChecksum(unsigned char* sentence, unsigned char size)'},1,10);s.File5=reshape({ '  void  uartMavlinkBufferInit(void)','  void __attribute__((__interrupt__,__auto_psv__)) _U1RXInterrupt(void)','  uint8_t  isFinite(float s)','  void  InitParameterInterface(void)','  void  protDecodeMavlink(void)','  uint16_t  MissionInterfaceResponse(uint8_t system_id, uint8_t component_id)','  uint16_t  ParameterInterfaceResponse(uint8_t system_id, uint8_t component_id)','  uint16_t  PackHeartBeat(uint8_t system_id, uint8_t component_id)','  uint16_t  PackTextMsg(uint8_t system_id, uint8_t component_id)','  uint16_t  PackRawIMU(uint8_t system_id, uint8_t component_id, mavlink_raw_imu_t mlRawIMUData ,uint32_t time_usec)','  uint16_t  PackGpsRawInt(uint8_t system_id, uint8_t component_id, mavlink_gps_raw_int_t mlRawGpsDataInt ,uint32_t time_usec)','  uint16_t  PackScaledPressure(uint8_t system_id, uint8_t component_id, mavlink_scaled_pressure_t mlAirData ,uint32_t time_usec)','  uint16_t  PackSysStatus(uint8_t system_id, uint8_t component_id, mavlink_sys_status_t mlSysStatus)','  char  sendQGCDebugMessage(const char * dbgMessage, char severity, unsigned char* bytesToAdd, char positionStart)','  void  TxN_Data_OverU1(uint16_t N)'},1,15);s.File6={ '  void  mavlinkInit(void)'};s.File7=reshape({ '  void  updateRawADCData(int16_t* adcData)','  void  updateAirData(float* airData)','  void  updateLoadData(uint8_t load, uint16_t mvPower)','  void  updateAttitude(float * attitudeData)','  void  getGSLocation(float* altLatLon)','  void  updateTimeStamp(uint32_t timeSt)','  void  updatePosition(float * posData)','  void  updatePilotConsole(uint16_t * pilData)','  void  updateDiagnosticFl(float* diagFl)','  void  updateDiagnosticSh(int16_t* diagSh)','  void  updateBias(float * biasData)','  void  updateSensorData(float* sens)','  uint8_t  isFixValid(void)','  void  updateSensorDiag(float* diag)'},1,14);s.File8=reshape({ '  void  gpsInit(void)','  void  gpsParse(uint8_t* dataStream)','  void  updateStatus(uint8_t* completeMessage)','  void  updatePositionData(uint8_t* completeMessage)','  void  updateVelocityData(uint8_t* completeMessage)','  void  updateTimeData(uint8_t* completeMessage)','  void  getGpsMainData(float* data)','  uint32_t  CRC32Value(int32_t i)','  uint32_t  CalculateBlockCRC32(uint32_t ulCount, uint8_t *ucBuffer)','  uint16_t  charsToUint16(uint8_t* data)','  uint32_t  charsToUint32(uint8_t* data)','  float  charsToFloat(uint8_t* data)','  double  charsToDouble(uint8_t* data)'},1,13);s.File9=reshape({ '  void  hilRead(unsigned char* hilChunk)','  void  hil_getRawRead(short * rawData)','  void  hil_getVned(float* vned)','  void  hil_getEuler(float* euler)','  void  hil_getRates(float* pqr)','  void  hil_getXYZ(float* xyz)',' unsigned int  hil_getTs(void)','  void  protDecodeHil(uint8_t* dataIn)'},1,8);s.File10=reshape({ '  void  cubeInit(void)','  void  getCubeData(short * cubeData)','  void  updateCubeData(void)','  int16_t  averageData(int16_t* theData, uint8_t count)',' unsigned short  write2Cube(unsigned short data2Send)','  void  __attribute__((interrupt, no_auto_psv)) _T5Interrupt(void)','  short  convert14BitToShort(short wordData)','  short  convert12BitToShort(short wordData)',' unsigned char  isCube16405(void)'},1,9);"  ORDERING=None  SampleTime=-1  MCHP_MASTERLINK=|  PinDigitalInput=[]  PinDigitalOutput=[]  PinAnalogInput=[]
      | AUAV_V3_TestSensors/Microchip Master
      | AUAV V3 Board
      | Busy Flag on D2 (RA6)
  negprotect : MATLAB Function  TreatAsAtomicUnit=on
  sqrt(x) : Outport
  wires:
  negprotect/1(zpVal) -> "[apUtils.c]"/1
  x/1 -> negprotect/1(val)
  "[apUtils.c]"/1 -> sqrt(x)/1

== system AUAV_V3_TestSensors/Position_and_Attitude_Filter/Attitude Complimentary Filter COG/Normalize Vector1/Norm/Subsystem3 ==
  x : Inport
  y : Inport  Port=2
  Embedded MATLAB Function : MATLAB Function  TreatAsAtomicUnit=on
  x dot y : Outport
  wires:
  y/1 -> Embedded MATLAB Function/2(y)
  x/1 -> Embedded MATLAB Function/1(x)
  Embedded MATLAB Function/1(xDoty) -> x dot y/1

== system AUAV_V3_TestSensors/Position_and_Attitude_Filter/Attitude Complimentary Filter COG/Normalize Vector2/Norm/Subsystem2 ==
  x : Inport
  "[apUtils.c]" : MCHP_Blockset/User Functions/C Function Call  ParseFilesChkbx=on  ListFunctions1=Custom Function  Function1=real32_T mySqrt(real32_T u1);  AddHeaderDeclaration=on  Function1Type=when block is updated (default)  FctReturnBlockOut=on  DataCollected="s.chksm=reshape({ '360325-Apr-2016 19:19:45','638502-Mar-2016 19:06:13','219625-Apr-2016 19:38:33','1593925-Apr-2016 19:41:14','3277826-Apr-2016 00:33:15','294426-Apr-2016 00:47:59','556001-Oct-2014 14:05:42','963201-Apr-2016 12:47:40','358819-Apr-2016 01:35:18','985925-Apr-2016 19:19:45'},1,10);s.File1=reshape({ '  float  myAtan2(float num, float denom)','  float  myPow(float x, float toTheN)','  float  mySqrt(float x)','  float  myAbs(float x)','  float  myAtan(float x)','  float  myAsin(float x)','  float  mySin(float x)','  float  myCos(float x)','  float  myTan(float x)','  float  myAcos(float x)','  float  myExp(float x)','  void  hugeDelay(void)','  void  smallDelay(void)','  void  tinyDelay(void)','  void  printToUart2(const char *fmt, ...)'},1,15);s.File2=reshape({ '  void  newCircBuffer(CBRef cB)','  void  freeCircBuffer(CBRef* cB)','  void  freeCircBuffer(CBRef* cB)',' unsigned int  getLength(CBRef cB)','  int  readHead(CBRef cB)','  int  readTail(CBRef cB)',' unsigned char  peak(CBRef cB)',' unsigned char  readFront(CBRef cB)',' unsigned char  writeBack(CBRef cB, unsigned char data)','  void  makeEmpty(CBRef cB)','  void  printCircBuf(CBRef cB)'},1,11);s.File3=reshape({ '  void  uartBufferInit(void)','  void  __attribute__((__interrupt__, no_auto_psv)) _U4RXInterrupt(void)','  void  getGPSRawData(unsigned char* gpsBuffer)',' unsigned char  isGPSNovatel(void)'},1,4);s.File4=reshape({ '  char  hex2char(char halfhex)','  float  degMinToDeg(unsigned char degrees, float minutes)',' unsigned char  gpsUbloxSeparate(unsigned char* outStream)','  void  gpsUbloxParse(void)','  void  getGpsUbloxMainData(float* data)','  char  gpSmbl(char symbl)',' unsigned char  myTokenizer(char* stringToTokenize, char token, char * returnToken)','  void  parseRMC(unsigned char* stream)','  void  parseGGA(unsigned char* stream)',' unsigned char  getChecksum(unsigned char* sentence, unsigned char size)'},1,10);s.File5=reshape({ '  void  uartMavlinkBufferInit(void)','  void __attribute__((__interrupt__,__auto_psv__)) _U1RXInterrupt(void)','  uint8_t  isFinite(float s)','  void  InitParameterInterface(void)','  void  protDecodeMavlink(void)','  uint16_t  MissionInterfaceResponse(uint8_t system_id, uint8_t component_id)','  uint16_t  ParameterInterfaceResponse(uint8_t system_id, uint8_t component_id)','  uint16_t  PackHeartBeat(uint8_t system_id, uint8_t component_id)','  uint16_t  PackTextMsg(uint8_t system_id, uint8_t component_id)','  uint16_t  PackRawIMU(uint8_t system_id, uint8_t component_id, mavlink_raw_imu_t mlRawIMUData ,uint32_t time_usec)','  uint16_t  PackGpsRawInt(uint8_t system_id, uint8_t component_id, mavlink_gps_raw_int_t mlRawGpsDataInt ,uint32_t time_usec)','  uint16_t  PackScaledPressure(uint8_t system_id, uint8_t component_id, mavlink_scaled_pressure_t mlAirData ,uint32_t time_usec)','  uint16_t  PackSysStatus(uint8_t system_id, uint8_t component_id, mavlink_sys_status_t mlSysStatus)','  char  sendQGCDebugMessage(const char * dbgMessage, char severity, unsigned char* bytesToAdd, char positionStart)','  void  TxN_Data_OverU1(uint16_t N)'},1,15);s.File6={ '  void  mavlinkInit(void)'};s.File7=reshape({ '  void  updateRawADCData(int16_t* adcData)','  void  updateAirData(float* airData)','  void  updateLoadData(uint8_t load, uint16_t mvPower)','  void  updateAttitude(float * attitudeData)','  void  getGSLocation(float* altLatLon)','  void  updateTimeStamp(uint32_t timeSt)','  void  updatePosition(float * posData)','  void  updatePilotConsole(uint16_t * pilData)','  void  updateDiagnosticFl(float* diagFl)','  void  updateDiagnosticSh(int16_t* diagSh)','  void  updateBias(float * biasData)','  void  updateSensorData(float* sens)','  uint8_t  isFixValid(void)','  void  updateSensorDiag(float* diag)'},1,14);s.File8=reshape({ '  void  gpsInit(void)','  void  gpsParse(uint8_t* dataStream)','  void  updateStatus(uint8_t* completeMessage)','  void  updatePositionData(uint8_t* completeMessage)','  void  updateVelocityData(uint8_t* completeMessage)','  void  updateTimeData(uint8_t* completeMessage)','  void  getGpsMainData(float* data)','  uint32_t  CRC32Value(int32_t i)','  uint32_t  CalculateBlockCRC32(uint32_t ulCount, uint8_t *ucBuffer)','  uint16_t  charsToUint16(uint8_t* data)','  uint32_t  charsToUint32(uint8_t* data)','  float  charsToFloat(uint8_t* data)','  double  charsToDouble(uint8_t* data)'},1,13);s.File9=reshape({ '  void  hilRead(unsigned char* hilChunk)','  void  hil_getRawRead(short * rawData)','  void  hil_getVned(float* vned)','  void  hil_getEuler(float* euler)','  void  hil_getRates(float* pqr)','  void  hil_getXYZ(float* xyz)',' unsigned int  hil_getTs(void)','  void  protDecodeHil(uint8_t* dataIn)'},1,8);s.File10=reshape({ '  void  cubeInit(void)','  void  getCubeData(short * cubeData)','  void  updateCubeData(void)','  int16_t  averageData(int16_t* theData, uint8_t count)',' unsigned short  write2Cube(unsigned short data2Send)','  void  __attribute__((interrupt, no_auto_psv)) _T5Interrupt(void)','  short  convert14BitToShort(short wordData)','  short  convert12BitToShort(short wordData)',' unsigned char  isCube16405(void)'},1,9);"  ORDERING=None  SampleTime=-1  MCHP_MASTERLINK=|  PinDigitalInput=[]  PinDigitalOutput=[]  PinAnalogInput=[]
      | AUAV_V3_TestSensors/Microchip Master
      | AUAV V3 Board
      | Busy Flag on D2 (RA6)
  negprotect : MATLAB Function  TreatAsAtomicUnit=on
  sqrt(x) : Outport
  wires:
  "[apUtils.c]"/1 -> sqrt(x)/1
  x/1 -> negprotect/1(val)
  negprotect/1(zpVal) -> "[apUtils.c]"/1

== system AUAV_V3_TestSensors/Position_and_Attitude_Filter/Attitude Complimentary Filter COG/Normalize Vector2/Norm/Subsystem3 ==
  x : Inport
  y : Inport  Port=2
  Embedded MATLAB Function : MATLAB Function  TreatAsAtomicUnit=on
  x dot y : Outport
  wires:
  Embedded MATLAB Function/1(xDoty) -> x dot y/1
  x/1 -> Embedded MATLAB Function/1(x)
  y/1 -> Embedded MATLAB Function/2(y)

== system AUAV_V3_TestSensors/Position_and_Attitude_Filter/Geod2LTP1/ECEF2LTP (UEN)/From Body to Universal1/Rotation Matrix from Long////Lat ==
  note: Calculate Coefficients of DCM Row-Wise
  long lat : Inport
  11 : Fcn  Expr=cos(u[1])*cos(u[2])
  12 : Fcn  Expr=sin(u[1])*cos(u[2])
  13 : Fcn  Expr=sin(u[2])
  21 : Fcn  Expr=-sin(u[1])
  22 : Fcn  Expr=cos(u[1])
  23 : Fcn  Expr=0
  31 : Fcn  Expr=-sin(u[2])*cos(u[1])
  32 : Fcn  Expr=-sin(u[1])*sin(u[2])
  33 : Fcn  Expr=cos(u[2])
  Mux2 : Mux  Inputs=9
  DCM : Outport
  wires:
  long lat/1 -> 21/1, 31/1, 12/1, 22/1, 32/1, 13/1, 23/1, 33/1, 11/1
  Mux2/1 -> DCM/1
  11/1 -> Mux2/1
  21/1 -> Mux2/2
  31/1 -> Mux2/3
  12/1 -> Mux2/4
  22/1 -> Mux2/5
  32/1 -> Mux2/6
  13/1 -> Mux2/7
  23/1 -> Mux2/8
  33/1 -> Mux2/9

== system AUAV_V3_TestSensors/Position_and_Attitude_Filter/Position Filter/BlendPosVel/2 FIlter Blend/Tustin Lowpass, Auto Initial Condition4 ==
  In1 : Inport
  Constant : Constant  Value=T
  Constant1 : Constant  Value=f
  Embedded MATLAB Function : MATLAB Function  TreatAsAtomicUnit=on
  Out1 : Outport
  wires:
  Constant/1 -> Embedded MATLAB Function/2(T)
  Constant1/1 -> Embedded MATLAB Function/3(f)
  Embedded MATLAB Function/1(y) -> Out1/1
  In1/1 -> Embedded MATLAB Function/1(u)

== system AUAV_V3_TestSensors/Position_and_Attitude_Filter/Position Filter/BlendPosVel/3D Filter/Filter1 ==
  In1 : Inport
  Discrete Zero-Pole : DiscreteZeroPole  Zeros=zerosd  Poles=polesd  Gain=gaind  SampleTime=SampleTime
  Out1 : Outport
  wires:
  In1/1 -> Discrete Zero-Pole/1
  Discrete Zero-Pole/1 -> Out1/1

== system AUAV_V3_TestSensors/Position_and_Attitude_Filter/Position Filter/BlendPosVel/3D Filter/Filter2 ==
  In1 : Inport
  Discrete Zero-Pole : DiscreteZeroPole  Zeros=zerosd  Poles=polesd  Gain=gaind  SampleTime=SampleTime
  Out1 : Outport
  wires:
  Discrete Zero-Pole/1 -> Out1/1
  In1/1 -> Discrete Zero-Pole/1

== system AUAV_V3_TestSensors/Position_and_Attitude_Filter/Position Filter/BlendPosVel/3D Filter/Filter3 ==
  In1 : Inport
  Discrete Zero-Pole : DiscreteZeroPole  Zeros=zerosd  Poles=polesd  Gain=gaind  SampleTime=SampleTime
  Out1 : Outport
  wires:
  In1/1 -> Discrete Zero-Pole/1
  Discrete Zero-Pole/1 -> Out1/1

== system AUAV_V3_TestSensors/Position_and_Attitude_Filter/Position Filter/BlendPosVel/CompFiltRate/1D Filter1 ==
  In1 : Inport
  Data Type Conversion1 : DataTypeConversion  OutDataTypeStr=single
  Data Type Conversion2 : DataTypeConversion  OutDataTypeStr=double
  Filter2 : Subsystem  mask(DiscretizedZeroPole){Zeros=zval, Poles=pval, Gain=kval, AbsTol=auto, SampleTime=TSample, method=tustin, Wc=1}
      mask prompts: Zeros "Zeros (enter in s-main:)"; Poles "Poles (enter in s-domain:)"; Gain "Gain (enter in s-domain:)"; AbsTol "Absolute tolerance:"; SampleTime "Sample time:"; Wc "Critical Frequency (Hz):"
      mask help: Continuous mask uses c2d to transform parameters onto the Discrete Zero-Pole block inside.
      mask init: same as AUAV_V3_TestSensors/Barometer_Driver/Baro Altimeter/Initial Baro Bias/Low Pass8
      mask TypeOptions method: zoh | foh | tustin | prewarp | matched
      mask Callback method: hidecrit
      mask Display:
      | droots(zeross,poless,gainss)
      | text( 0.5, 1.0, method, 'verticalAlignment','top')
  Out1 : Outport
  wires:
  Data Type Conversion1/1 -> Out1/1
  Data Type Conversion2/1 -> Filter2/1(In1)
  In1/1 -> Data Type Conversion2/1
  Filter2/1(Out1) -> Data Type Conversion1/1

== system AUAV_V3_TestSensors/Position_and_Attitude_Filter/Position Filter/BlendPosVel/CompFiltRate1/1D Filter1 ==
  In1 : Inport
  Data Type Conversion1 : DataTypeConversion  OutDataTypeStr=single
  Data Type Conversion2 : DataTypeConversion  OutDataTypeStr=double
  Filter2 : Subsystem  mask(DiscretizedZeroPole){Zeros=zval, Poles=pval, Gain=kval, AbsTol=auto, SampleTime=TSample, method=tustin, Wc=1}
      mask prompts: Zeros "Zeros (enter in s-main:)"; Poles "Poles (enter in s-domain:)"; Gain "Gain (enter in s-domain:)"; AbsTol "Absolute tolerance:"; SampleTime "Sample time:"; Wc "Critical Frequency (Hz):"
      mask help: Continuous mask uses c2d to transform parameters onto the Discrete Zero-Pole block inside.
      mask init: same as AUAV_V3_TestSensors/Barometer_Driver/Baro Altimeter/Initial Baro Bias/Low Pass8
      mask TypeOptions method: zoh | foh | tustin | prewarp | matched
      mask Callback method: hidecrit
      mask Display:
      | droots(zeross,poless,gainss)
      | text( 0.5, 1.0, method, 'verticalAlignment','top')
  Out1 : Outport
  wires:
  Data Type Conversion1/1 -> Out1/1
  Data Type Conversion2/1 -> Filter2/1(In1)
  In1/1 -> Data Type Conversion2/1
  Filter2/1(Out1) -> Data Type Conversion1/1

== system AUAV_V3_TestSensors/Position_and_Attitude_Filter/Position Filter/BlendPosVel/CompRateOnly/1D Filter1 ==
  In1 : Inport
  Data Type Conversion1 : DataTypeConversion  OutDataTypeStr=single
  Data Type Conversion2 : DataTypeConversion  OutDataTypeStr=double
  Filter2 : Subsystem  mask(DiscretizedZeroPole){Zeros=zval, Poles=pval, Gain=kval, AbsTol=auto, SampleTime=TSample, method=tustin, Wc=1}
      mask prompts: Zeros "Zeros (enter in s-main:)"; Poles "Poles (enter in s-domain:)"; Gain "Gain (enter in s-domain:)"; AbsTol "Absolute tolerance:"; SampleTime "Sample time:"; Wc "Critical Frequency (Hz):"
      mask help: Continuous mask uses c2d to transform parameters onto the Discrete Zero-Pole block inside.
      mask init: same as AUAV_V3_TestSensors/Barometer_Driver/Baro Altimeter/Initial Baro Bias/Low Pass8
      mask TypeOptions method: zoh | foh | tustin | prewarp | matched
      mask Callback method: hidecrit
      mask Display:
      | droots(zeross,poless,gainss)
      | text( 0.5, 1.0, method, 'verticalAlignment','top')
  Out1 : Outport
  wires:
  Data Type Conversion1/1 -> Out1/1
  Data Type Conversion2/1 -> Filter2/1(In1)
  In1/1 -> Data Type Conversion2/1
  Filter2/1(Out1) -> Data Type Conversion1/1

== system AUAV_V3_TestSensors/Sensor_Data_Adapter/Sensor Suite/Low Pass Filtering,Temperature Compensation and Calibration/Baro Altimeter/Compute Barometric Height ==
  Base Height (m) : Inport
  Base Pressure (Pa) : Inport  Port=2
  Baro (Pa) : Inport  Port=3
  Constant2 : Constant  Value=baseTemp/(-LapseRate)  OutDataTypeStr=single
  Constant3 : Constant  Value=9.350253e-2  OutDataTypeStr=single
  Constant4 : Constant  Value=-1.888933e-1  OutDataTypeStr=single
  Constant5 : Constant  Value=2.180313e-5  OutDataTypeStr=single
  Divide : Product  Inputs=*/  OutDataTypeStr=single
  Divide{1..4} (4 alike) : Product  OutDataTypeStr=single
  Length Conversion : aerolibconvert2/Length Conversion  IU=ft  OU=m
  Sum1 : Sum  Inputs=|++  OutDataTypeStr=single
  Sum2 : Sum  Inputs=|+-  OutDataTypeStr=single
  Sum3 : Sum  Inputs=3  OutDataTypeStr=single
  "Altitude, m" : Outport
  wires:
  Length Conversion/1 -> Sum1/1
  Sum2/1 -> Divide/1
  Sum1/1 -> "Altitude, m"/1
  Divide3/1 -> Length Conversion/1
  Constant2/1 -> Divide3/2
  Sum3/1 -> Divide3/1
  Constant5/1 -> Sum3/3
  Divide2/1 -> Sum3/2
  Divide1/1 -> Sum3/1
  Constant4/1 -> Divide2/2
  Constant3/1 -> Divide1/2
  Divide4/1 -> Divide1/1  "x^2"
  Divide/1 -> Divide2/1, Divide4/1, Divide4/2  "x"
  Base Pressure (Pa)/1 -> Divide/2, Sum2/2
  Base Height (m)/1 -> Sum1/2
  Baro (Pa)/1 -> Sum2/1
